simulink model "parent_model"  (R2024a)
settings: Solver=VariableStepAuto  StartTime=0.0  StopTime=50  RelTol=1e-3
libraries: sharedtransform x1
settings Model: Creator=aryam  LastModifiedBy=ashis
settings RTWCC: GPUComputeCapability=3.5

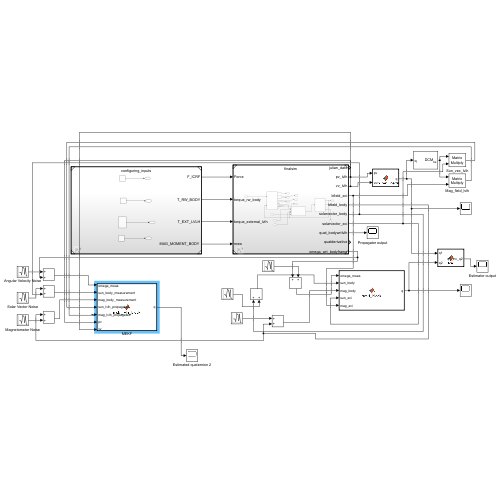
[thumbnail: Simulink's stored preview of the top-level diagram]
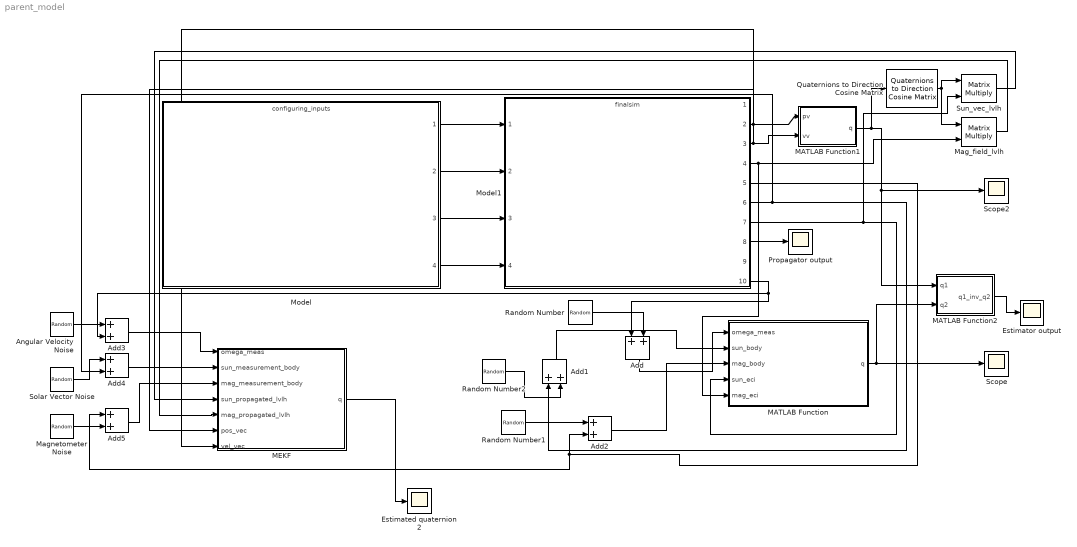
== system parent_model ==
  Add{,1..5} (6 alike) : Sum
  Angular Velocity Noise : RandomNumber  Variance=0  SampleTime=0.1
  Estimated quaternion 2 : Scope
  Estimator output : Scope
  MATLAB Function : MATLAB Function  TreatAsAtomicUnit=on
  MATLAB Function1 : MATLAB Function  TreatAsAtomicUnit=on
  MATLAB Function2 : MATLAB Function  TreatAsAtomicUnit=on
  MEKF : MATLAB Function  TreatAsAtomicUnit=on
  Mag_field_lvlh : Product  Multiplication=Matrix(*)
  Magnetometer Noise : RandomNumber  Variance=0  SampleTime=0.1
  Model : ModelReference  ModelNameDialog=configuring_inputs.slx  SimulationMode=Normal  ModelReferenceVersion=2.3
  Model1 : ModelReference  ModelNameDialog=finalsim.slx  SimulationMode=Normal  ModelReferenceVersion=2.1
  Propagator output : Scope
  Quaternions to Direction Cosine Matrix : sharedtransform/Quaternions to  Direction Cosine Matrix  aMode=aMode
      settings: LibrarySourceBlock=|
      | aerolibtransform2/Quaternions to
      | Direction Cosine Matrix
  Random Number : RandomNumber  Mean=0.1  Variance=0.01  SampleTime=0.1
  Random Number1 : RandomNumber  Mean=1e-6  Variance=2e-10  SampleTime=0.1  VectorParams1D=off
  Random Number2 : RandomNumber  Variance=0.3  SampleTime=0.1  VectorParams1D=off
  Scope : Scope
  Scope2 : Scope
  Solar Vector Noise : RandomNumber  Variance=0  SampleTime=0.1  VectorParams1D=off
  Sun_vec_lvlh : Product  Multiplication=Matrix(*)
  wires:
  Model/1 -> Model1/1
  Model/2 -> Model1/2
  Model/3 -> Model1/3
  Model/4 -> Model1/4
  Model1/10 -> Add3/2, Add/1
  Model1/7 -> Sun_vec_lvlh/2, MATLAB Function/4(sun_eci)
  Model1/6 -> Add4/2, Add1/1
  Model1/5 -> Add5/1, Add2/2
  MATLAB Function/1(q) -> MATLAB Function2/2(q2), Scope/1
  Model1/8 -> Propagator output/1
  Model1/2 -> MEKF/6(pos_vec), MATLAB Function1/1(pv)
  Model1/3 -> MEKF/7(vel_vec), MATLAB Function1/2(vv)
  MATLAB Function1/1(q) -> Quaternions to Direction Cosine Matrix/1, MATLAB Function2/1(q1), Scope2/1
  MATLAB Function2/1(q1_inv_q2) -> Estimator output/1
  Add/1 -> MATLAB Function/1(omega_meas)
  Random Number/1 -> Add/2
  Random Number1/1 -> Add2/1
  Model1/4 -> Mag_field_lvlh/2, MATLAB Function/5(mag_eci)
  Add2/1 -> MATLAB Function/3(mag_body)
  Random Number2/1 -> Add1/2
  Add1/1 -> MATLAB Function/2(sun_body)
  Quaternions to Direction Cosine Matrix/1 -> Sun_vec_lvlh/1, Mag_field_lvlh/1
  Sun_vec_lvlh/1 -> MEKF/4(sun_propagated_lvlh)
  Mag_field_lvlh/1 -> MEKF/5(mag_propagated_lvlh)
  MEKF/1(q) -> Estimated quaternion 2/1
  Angular Velocity Noise/1 -> Add3/1
  Add3/1 -> MEKF/1(omega_meas)
  Solar Vector Noise/1 -> Add4/1
  Add4/1 -> MEKF/2(sun_measurement_body)
  Magnetometer Noise/1 -> Add5/2
  Add5/1 -> MEKF/3(mag_measurement_body)

== matlab function parent_model/MATLAB Function1 ==
  data: pv input; q output; vv input
function q = q_lvlh_wrt_inertial(pv, vv)
    
    % Calculate the LVLH frame axes
    z = -pv / norm(pv);               % Local vertical (negative of position vector)
    y = cross(z, vv) / norm(cross(z, vv));  % Local horizontal (cross product of z and velocity)
    x = cross(y, z);                  % Cross product of y and z to get x axis

    % Construct the direction cosine matrix
    m = [x, y, z]';

    % Convert DCM to quaternion
    q = rotm2quat(m);
    qres = [q(1), q(2), q(3), q(4)];

    q = qres;    
    % MATLAB's dcm2quat returns quaternions in the form [w x y z]
    % Some conventions use [x y z w], ensure your convention matches your needs
end

== matlab function parent_model/MATLAB Function ==
  settings: updateMethod=DISCRETE
  data: omega_meas input; q output; sun_body input; mag_body input; sun_eci input; mag_eci input
function q  = mekf_block(omega_meas, sun_body, mag_body, sun_eci, mag_eci)
    %#codegen

    persistent mekf
    if isempty(mekf)
        R_input = diag([0.0001, 0.0001, 0.0001, 0.0001, 0.0001, 0.0001]); % Example values
        P_start = eye(6); % Example values
        x_init = [0;0;0;0.1;0.1;0.1];
        dt = 0.1; % Example time step
        std_dev_process = [0.01, 0.01, 0.01, 0.01, 0.01, 0.01]; % Example values
        mekf = MEKF(R_input, P_start, x_init, dt, std_dev_process);
    end

    % Reset the MEKF object if required
    if norm(mekf.del_x (1:3)) > pi/18
        mekf.reset();
    end

    

    % Update the measurement
    zk = [sun_body; mag_body];

    mekf = measurement_update(mekf, zk, sun_eci, mag_eci);

    % Predict the state
    mekf = predict_state(mekf, omega_meas);
    % Output the estimated quaternion
    q_est = mekf.q_est;
    temp = q_est;
    q = q_est';
    %q = quaternion(q_est');
end

== matlab function parent_model/MATLAB Function2 ==
  data: q1 input; q1_inv_q2 output; q2 input
function q1_inv_q2 = fcn(q1, q2)

    quat1_inv = [q1(1), -q1(2), -q1(3), -q1(4)];

    q1_inv_q2 = quatmultiply(quat1_inv, q2);

    q1_inv_q2 = [q1_inv_q2(1), q1_inv_q2(2), q1_inv_q2(3), q1_inv_q2(4)];
end

== matlab function parent_model/MEKF ==
  settings: updateMethod=DISCRETE
  data: omega_meas input; q output; sun_measurement_body input; mag_measurement_body input; sun_propagated_lvlh input; mag_propagated_lvlh input; pos_vec input; vel_vec input
function q  = mekf_lvlh_block(omega_meas, sun_measurement_body, mag_measurement_body, sun_propagated_lvlh, mag_propagated_lvlh, pos_vec, vel_vec)

    % Add this to the MATLAB function block in Simulink
    
    % Inputs:(All inputs need to be as column vectors)
    %   omega_meas : Measured angular velocity in body frame
    %   sun_measurement_body: Unit solar vector measured in body frame 
    %   mag_measurement_body: Magnetic field vector measured in body frame
    %   sun_propagated_body: Unit solar vector in orbit(lvlh) frame, from propagator
    %   mag_propagated_body: Magnetic field vector in orbit(lvlh) frame, from propagator
    %   pos_vec is the position vector in inertial frame, from propagator
    %   vel_vec is the velocity vector in inertial frame, from propagator
    
    % Output: 
    %   q: quaternion of the body frame w.r.t. the orbit frame as a column vector

    % Persistent variable means that the function remembers this variable between function calls
    persistent mekf_new

    if isempty(mekf_new)

        % Initialise an instance of the mekf_new class
        % These values can be edited once we have done sensor modelling 
        % And tested various values

        R_input = diag([0.005, 0.005, 0.005, 0.0007, 0.0007, 0.0007]); % Example values
        P_start = eye(6); % Example values
        x_init = [0;0;0;0.0;0.0;0.0]; %% The last three elements to be replaced by the GYRO BIAS VECTOR *******
        dt = 0.1; % Example time step
        std_dev_process = [0.01, 0.01, 0.01, 0.01, 0.01, 0.01]; % Example values

        mekf_new = MEKF_lvlh(R_input, P_start, x_init, dt, std_dev_process);
    end


    % Reset the MEKF object if required
    if norm(mekf_new.del_x (1:3)) > pi/18 % choosing when we want to reset the del_x and quaternion; this can be changed too
        mekf_new.reset();
    end

    
    % Measurement update 
    zk = [sun_measurement_body; mag_measurement_body];
    mekf_new = measurement_update(mekf_new, zk, sun_propagated_lvlh, mag_propagated_lvlh);
    
    % Predict the state
    mekf_new = predict_state(mekf_new, omega_meas, pos_vec, vel_vec);
    

    q = mekf_new.q_est; % The estimate of the quaternion of body frame w.r.t orbit frame
end
